simulink model "LineFollower"  (R2016a)
settings: Solver=FixedStepAuto  SolverMode=SingleTasking  StartTime=0.0  StopTime=inf  RelTol=1e-3
libraries: arduinolib x9
settings Model: SimulationMode=external  ExtModeTrigDuration=2  Creator=areej_ofamech  LastModifiedBy=areej_ofamech
settings OptimizationCC: OptimizeModelRefInitCode=on  LifeSpan=Inf  MaxStackSize=64
settings HardwareCC: ProdBitPerInt=16  ProdBitPerPointer=16  ProdLargestAtomicFloat=None  ProdWordSize=8  ProdHWDeviceType=Atmel->AVR
settings RTWCC: SystemTargetFile=ert.tlc  HardwareBoard=Arduino Uno  TemplateMakefile=ert_default_tmf  GenerateReport=on  Toolchain=Arduino AVR v1.6.1  BuildConfiguration=Faster Runs  IncludeHyperlinkInReport=on  LaunchReport=on  GenerateTraceInfo=on  GenerateTraceReport=on  GenerateTraceReportSl=on  GenerateTraceReportSf=on  GenerateTraceReportEml=on
settings CodeAppCC: ForceParamTrailComments=on  IgnoreCustomStorageClasses=off  OperatorAnnotations=on  SimulinkDataObjDesc=on  SFDataObjDesc=on  MATLABFcnDesc=on  MangleLength=10  InsertBlockDesc=on  MATLABSourceComments=on
settings ERTTargetCC: SupportContinuousTime=on  SupportVariableSizeSignals=on  ExtMode=on  ExtModeTransport=3  ExtModeMexFile=ext_serial_win32_comm_rtt  ExtModeMexArgs=0 6 115200

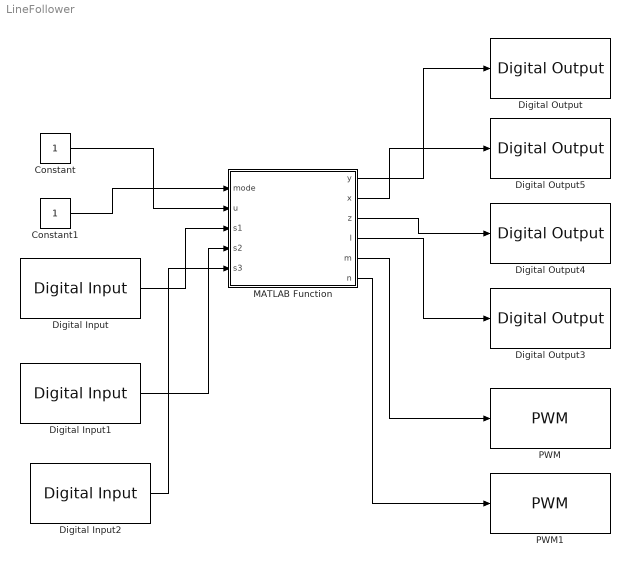
== system LineFollower ==
  Constant : Constant
  Constant1 : Constant
  Digital Input : arduinolib/Digital Input  pinNumber=3  sampleTime=1  blockPlatform=arduino
  Digital Input1 : arduinolib/Digital Input  pinNumber=4  sampleTime=1  blockPlatform=arduino
  Digital Input2 : arduinolib/Digital Input  pinNumber=5  sampleTime=1  blockPlatform=arduino
  Digital Output : arduinolib/Digital Output  pinNumber=8  blockPlatform=arduino
  Digital Output3 : arduinolib/Digital Output  pinNumber=13  blockPlatform=arduino
  Digital Output4 : arduinolib/Digital Output  pinNumber=12  blockPlatform=arduino
  Digital Output5 : arduinolib/Digital Output  pinNumber=9  blockPlatform=arduino
  MATLAB Function : MATLAB Function  TreatAsAtomicUnit=on
  PWM : arduinolib/PWM  pinNumber=10  blockPlatform=arduino
  PWM1 : arduinolib/PWM  pinNumber=11  blockPlatform=arduino
  wires:
  MATLAB Function/1(y) -> Digital Output/1
  MATLAB Function/2(x) -> Digital Output5/1
  MATLAB Function/3(z) -> Digital Output4/1
  MATLAB Function/4(l) -> Digital Output3/1
  Constant/1 -> MATLAB Function/2(u)
  MATLAB Function/5(m) -> PWM/1
  MATLAB Function/6(n) -> PWM1/1
  Digital Input/1 -> MATLAB Function/3(s1)
  Digital Input1/1 -> MATLAB Function/4(s2)
  Constant1/1 -> MATLAB Function/1(mode)
  Digital Input2/1 -> MATLAB Function/5(s3)

== matlab function LineFollower/MATLAB Function ==
  data: mode input; u input; y output; x output; z output; l output; m output; n output; s1 input; s2 input; s3 input
function [y,x,z,l,m,n] = fcn(mode ,u, s1,s2,s3)
y=0;
x=0;
z=0;
l=0;
m=80;
n=80;
%Manual
if (mode ==0)
    switch u
        case 0
            %forward
            y=1;
            x=0;
            z=0;
            l=1;
            m=80;
            n=80;
            
        case 1
            %backward
            y=0;
            x=1;
            z=1;
            l=0;
            m=80;
            n=80;
            
        case 2
            %right
            y=1;
            x=0;
            z=0;
            l=1;
            m=60;
            n=80;
        case 3
            %left
            y=1;
            x=0;
            z=0;
            l=1;
            m=80;
            n=60;
    end
    %Line
elseif (mode ==1)
    %right
    if(s1 == 0 && s2 ==1 && s3 ==1)
        y=1;
        x=0;
        z=0;
        l=1;
        m=80;
        n=50;
        %forward
    elseif(s1 ==0 && s2 ==0 && s3 ==0)
        y=1;
        x=0;
        z=0;
        l=1;
        m=80;
        n=80;
        %left
    elseif(s1 == 1 && s2 ==1 && s3 ==0)
        y=1;
        x=0;
        z=0;
        l=1;
        m=50;
        n=80;
    end
else
    y=0;
    x=0;
    z=0;
    l=0;
end
end
